simulink model "Problem_6"  (R2022a)
settings: Solver=FixedStepAuto  StartTime=0.0  StopTime=20  FixedStep=0.0001  RelTol=1e-3
libraries: simulink x1
settings Model: Creator=Shocky  LastModifiedBy=Shocky

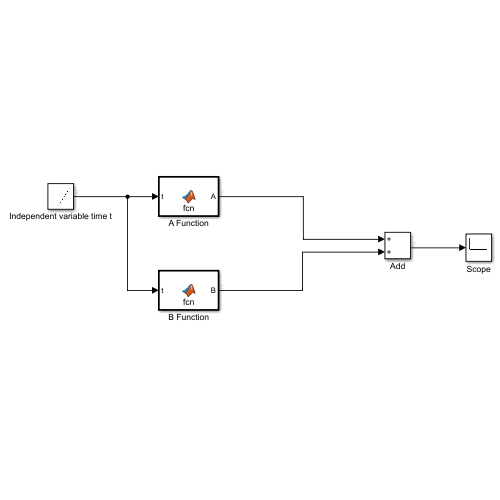
[thumbnail: Simulink's stored preview of the top-level diagram]
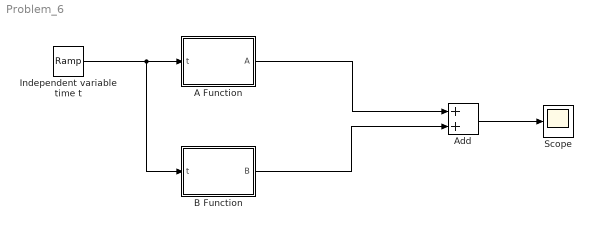
== system Problem_6 ==
  A Function : MATLAB Function  TreatAsAtomicUnit=on
  Add : Sum
  B Function : MATLAB Function  TreatAsAtomicUnit=on
  Independent variable time t : simulink/Sources/Ramp  slope=1  start=0  InitialOutput=0
  Scope : Scope
  wires:
  Independent variable time t/1 -> B Function/1(t), A Function/1(t)
  A Function/1(A) -> Add/1
  B Function/1(B) -> Add/2
  Add/1 -> Scope/1

== matlab function Problem_6/A Function ==
  data: t input; A output
function A= fcn(t)
Gamma=254321; 
A=2.*sin(Gamma./30000.*t)+3.*cos(t);
end

== matlab function Problem_6/B Function ==
  data: t input; B output
function B = fcn(t)
B=20.*exp(-0.5.*t);
end
